simulink model "Pendulum_Plant"  (R2023a)
settings: Solver=ode4  StartTime=0.0  StopTime=5  FixedStep=0.001  RelTol=1e-3
settings Model: Creator=Fasih  LastModifiedBy=Fasih

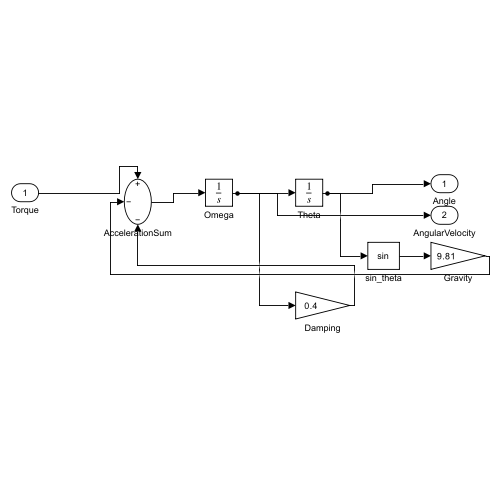
[thumbnail: Simulink's stored preview of the top-level diagram]
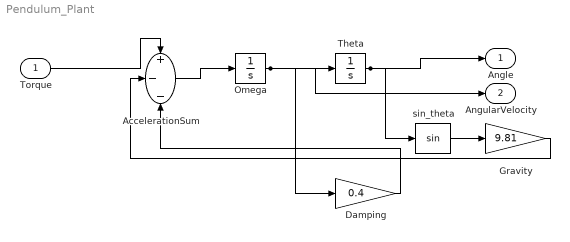
== system Pendulum_Plant ==
  Torque : Inport
  AccelerationSum : Sum  Inputs=+--
  Damping : Gain  Gain=0.4
  Gravity : Gain  Gain=9.81
  Omega : Integrator
  Theta : Integrator
  sin_theta : Trigonometry
  Angle : Outport
  AngularVelocity : Outport  Port=2
  wires:
  Torque/1 -> AccelerationSum/1
  AccelerationSum/1 -> Omega/1
  Omega/1 -> Theta/1, AngularVelocity/1, Damping/1
  Theta/1 -> Angle/1, sin_theta/1
  sin_theta/1 -> Gravity/1
  Gravity/1 -> AccelerationSum/2
  Damping/1 -> AccelerationSum/3
